simulink model "Temperature_Control_System"  (R2023a)
settings: Solver=VariableStepAuto  StartTime=0.0  StopTime=10.0  RelTol=1e-3
values from neighbouring files (symbols this model uses):
  k = 3    [Tem_control_system.m]
settings Model: Creator=Mass  LastModifiedBy=Mass

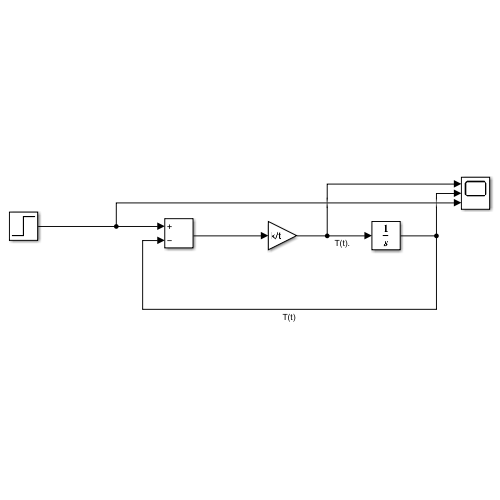
[thumbnail: Simulink's stored preview of the top-level diagram]
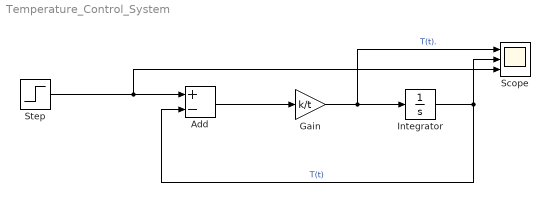
== system Temperature_Control_System ==
  Add : Sum  Inputs=+-
  Gain : Gain  Gain=k/t
  Integrator : Integrator
  Scope : Scope  NumInputPorts=3
  Step : Step  Time=3  After=20  SampleTime=0
  wires:
  Step/1 -> Scope/3, Add/1
  Add/1 -> Gain/1
  Gain/1 -> Scope/1, Integrator/1  "T(t)."
  Integrator/1 -> Scope/2, Add/2  "T(t)"
